simulink library "dspmisc"  (Simulink 8.0)
settings: Solver=ode45  SolverMode=SingleTasking  StartTime=0.0  StopTime=10.0  RelTol=1e-3
values from neighbouring files (symbols this model uses):
  D = D + B    [rebuffer_delay.m]
undefined symbols (not defined in the file or in its folder): get
libraries: dspsigattribs x2, dspsnks4 x1, dspmtrx3 x1, dspmathops x1, dspobslib x1, simulink x1
settings Model: Creator=mani  LastModifiedBy=lij  ExtModeAutoUpdateStatusClock=off

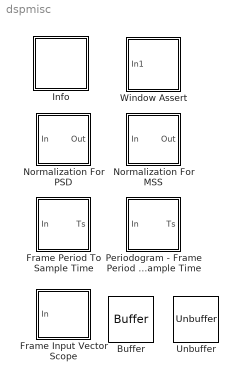
== system dspmisc ==
  Buffer : Buffer
  Frame Input Vector Scope : Subsystem
  Frame Period To Sample Time : Subsystem
  Info : Subsystem
      settings: OpenFcn=web(dspdhelp('dsp'), '-helpbrowser');
      mask Type: Info
      mask Display: disp('Info')
  Normalization For MSS : Subsystem
  Normalization For PSD : Subsystem
  Periodogram - Frame Period To Sample Time : Subsystem
  Unbuffer : Unbuffer
  Window Assert : Subsystem  mask{winsize=512, decimat=16, tol=10e-16}
      mask prompts: winsize "Window size:"; decimat "Decimation:"; tol "Tolerance"

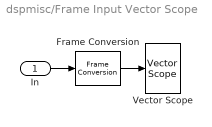
== system dspmisc/Frame Input Vector Scope ==
  In : Inport
  Frame Conversion : FrameConversion
  Vector Scope : dspsnks4/Vector Scope  ScopeProperties=on  Domain=Time  HorizSpan=1  DisplayProperties=off  AxisGrid=on  Memory=off  FrameNumber=on  AxisLegend=off  AxisZoom=off  OpenScopeAtSimStart=on  OpenScopeImmediately=off  FigPos=get(0,'defaultfigureposition')  AxisProperties=off  XUnits=Hertz  XRange=[0...Fs/2]  InheritXIncr=on  XIncr=1  XLabel=Time  XLimit=Auto  XMin=0  XMax=1  XStart=0  YUnits=dB  YLabel=Amplitude  LineProperties=off  XAxisParamsVer=6.9
      settings: YMin=-10  YMax=10
  wires:
  Frame Conversion/1 -> Vector Scope/1
  In/1 -> Frame Conversion/1

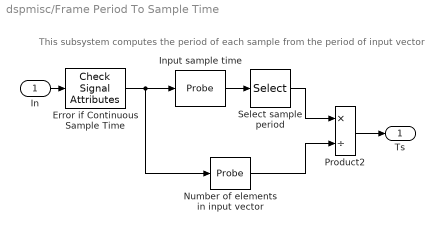
== system dspmisc/Frame Period To Sample Time ==
  note: This subsystem computes the period of each sample
      | from the period of input vector
  In : Inport
  Error if Continuous Sample Time : dspsigattribs/Check Signal Attributes  SystemSampleTime=-1  SigAttribCheckMethod=Matches attributes exactly  Complexity=Ignore  Frame=Ignore  DimsCheckMethod=Ignore  Dimensions=Row vector (2-D)  DatatypeCheckMethod=Ignore  DatatypeGeneral=Boolean  DtypeFloatSpecific=Any floating-point  DtypeFixedSpecific=Any fixed-point  DtypeIntSpecific=Any integer  SampleMode=Continuous
  Input sample time : Probe  ProbeWidth=off  ProbeComplexSignal=off  ProbeSampleTimeDataType=Same as input
  Number of elements in input vector : Probe  ProbeSampleTime=off  ProbeComplexSignal=off  ProbeWidthDataType=Same as input
  Product2 : Product  Inputs=*/  SaturateOnIntegerOverflow=on  InputSameDT=on  OutDataTypeStr=Inherit: Same as first input
  Select sample period : Selector  InputPortWidth=2  IndexOptions=Index vector (dialog)  Indices=[1]  OutputSizes=1
  Ts : Outport
  wires:
  In/1 -> Error if Continuous Sample Time/1
  Number of elements in input vector/1 -> Product2/2
  Product2/1 -> Ts/1
  Input sample time/1 -> Select sample period/1
  Select sample period/1 -> Product2/1
  Error if Continuous Sample Time/1 -> Number of elements in input vector/1, Input sample time/1

== system dspmisc/Info ==

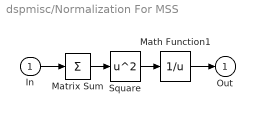
== system dspmisc/Normalization For MSS ==
  In : Inport
  Math Function1 : Math  Operator=reciprocal  SaturateOnIntegerOverflow=on
  Matrix Sum : Sum  Inputs=+  CollapseMode=Specified dimension
  Square : Math  Operator=square  SaturateOnIntegerOverflow=on
  Out : Outport
  wires:
  Square/1 -> Math Function1/1
  Matrix Sum/1 -> Square/1
  In/1 -> Matrix Sum/1
  Math Function1/1 -> Out/1

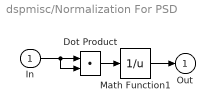
== system dspmisc/Normalization For PSD ==
  In : Inport
  Dot Product : DotProduct  OutDataTypeStr=Inherit: Inherit via internal rule
  Math Function1 : Math  Operator=reciprocal  SaturateOnIntegerOverflow=on
  Out : Outport
  wires:
  In/1 -> Dot Product/2, Dot Product/1
  Math Function1/1 -> Out/1
  Dot Product/1 -> Math Function1/1

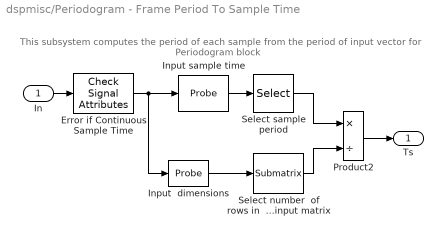
== system dspmisc/Periodogram - Frame Period To Sample Time ==
  note: This subsystem computes the period of each sample
      | from the period of input vector for Periodogram block
  In : Inport
  Error if Continuous Sample Time : dspsigattribs/Check Signal Attributes  SystemSampleTime=-1  SigAttribCheckMethod=Matches attributes exactly  Complexity=Ignore  Frame=Ignore  DimsCheckMethod=Ignore  Dimensions=Row vector (2-D)  DatatypeCheckMethod=Ignore  DatatypeGeneral=Boolean  DtypeFloatSpecific=Any floating-point  DtypeFixedSpecific=Any fixed-point  DtypeIntSpecific=Any integer  SampleMode=Continuous
  Input  dimensions : Probe  ProbeWidth=off  ProbeSampleTime=off  ProbeComplexSignal=off  ProbeSignalDimensions=on  ProbeDimensionsDataType=Same as input
  Input sample time : Probe  ProbeWidth=off  ProbeComplexSignal=off  ProbeSampleTimeDataType=Same as input
  Product2 : Product  Inputs=*/  SaturateOnIntegerOverflow=on  InputSameDT=on  OutDataTypeStr=Inherit: Same as first input
  Select sample period : Selector  InputPortWidth=2  IndexOptions=Index vector (dialog)  Indices=[1]  OutputSizes=1
  Select number  of rows in  input matrix : dspmtrx3/Submatrix  RowSpan=One row  RowStartMode=First  RowStartIndex=1  RowEndMode=Last  RowEndIndex=1  ColSpan=All columns  ColStartMode=First  ColStartIndex=1  ColEndMode=Last  ColEndIndex=1
  Ts : Outport
  wires:
  Product2/1 -> Ts/1
  Select number  of rows in  input matrix/1 -> Product2/2
  Input sample time/1 -> Select sample period/1
  In/1 -> Error if Continuous Sample Time/1
  Input  dimensions/1 -> Select number  of rows in  input matrix/1
  Select sample period/1 -> Product2/1
  Error if Continuous Sample Time/1 -> Input  dimensions/1, Input sample time/1

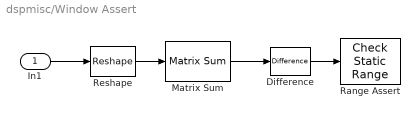
== system dspmisc/Window Assert ==
  In1 : Inport
  Difference : dspmathops/Difference  dim=Columns  Dimension=1  roundingMode=Floor  overflowMode=off
  Matrix Sum : dspobslib/Matrix Sum  Dim=Rows  roundingMode=Floor  overflowMode=off
  Range Assert : simulink/Model Verification/Check  Static Range  Description=-tol <= u <= tol  SystemSampleTime=-1  max=tol  max_included=on  min=-tol  min_included=on  enabled=on  stopWhenAssertionFail=on  export=off  icon=graphic
  Reshape : Reshape  OutputDimensionality=Customize  OutputDimensions=[decimat, winsize/decimat]
  wires:
  In1/1 -> Reshape/1
  Reshape/1 -> Matrix Sum/1
  Matrix Sum/1 -> Difference/1
  Difference/1 -> Range Assert/1
